simulink model "MARS"  (R2022a)
settings: Solver=VariableStepAuto  StartTime=0.0  StopTime=inf  RelTol=1e-3
model workspace (MAT data in the model file):
  T0 = -23.4
  h_trop = 7
  ingenuityParams : object (value not decoded)
values from neighbouring files (symbols this model uses):
  ingenuityParams =     [marsBatParam.mat]
undefined symbols (not defined in the file or in its folder): body, collective1, collective2, duration, ingenuity, leg1, leg2, leg3, leg4, link_name, model_name, rotor1, rotor2, solarPanel, world_pose
libraries: fl_lib x35, robotgazebolib x31, nesl_utility x12, ee_lib x11, slpidlib x3, sharedtransform x2, simulink x1, shared6dof x1, aerolibwind2 x1
(part 3 of 3)

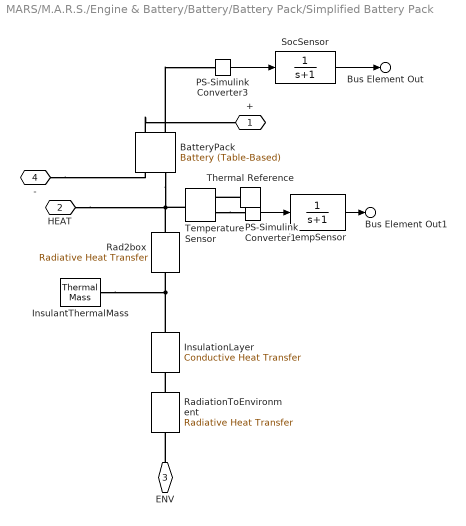
== system MARS/M.A.R.S./Engine & Battery/Battery/Battery Pack/Simplified Battery Pack ==
  BatteryPack : ee_lib/Sources/Battery (Table-Based)  SOC_vec=ingenuityParams.battery.cell.SOCvec  T_dependence=ee.enum.temperature_dependence.yes  prm_dir=ee.enum.battery.prm_dir.noCurrentDirectionality  T_vec=ingenuityParams.battery.cell.Tvec degC  V0_mat=ingenuityParams.battery.cell.V0_TLU*ingenuityParams.battery.numSeriesCells V  V0_vec=[3.1, 3.27, 3.31, 3.5] V  R0_mat=ingenuityParams.battery.cell.R0_TLU*ingenuityParams.battery.numSeriesCells/ingenuityParams.battery.numParallelStrings Ohm  R0_vec=[.015, .017, .012, .013] Ohm  R0_dis_mat=[.03, .015, .002; .04, .017, .008; .039, .012, .006; .027, .013, .021] Ohm  R0_dis_vec=[.015, .017, .012, .013] Ohm  R0_ch_mat=[.03, .015, .002; .04, .017, .008; .039, .012, .006; .027, .013, .021] Ohm  R0_ch_vec=[.015, .017, .012, .013] Ohm  AH=ingenuityParams.battery.cell.AH_TLU*ingenuityParams.battery.numParallelStrings A*hr  prm_leak=ee.enum.battery.prm_leak.disabled  Rleak_vec=[8000, 7000, 6000] Ohm  Rleak=7e3 Ohm  extrapolation_option=simscape.enum.extrapolation.nearest  SOC_port=ee.enum.enable.yes  V_range=[0, inf] V  prm_dyn=ee.enum.battery.prm_dyn.off  R1_mat=[.089, .076, .01; .042, .022, .099; .019, .007, .002; .051, .043, .029] Ohm  R1_vec=[.076, .022, .007, .043] Ohm  tau1_mat=[44, 148, 235; 93, 110, 1000; 19, 27, 133; .5, 22, 3] s  tau1_vec=[148, 110, 27, 22] s  R2_mat=[.014, .382, .407; .028, .006, .007; .014, .007, .006; .333, .956, .912] Ohm  R2_vec=[.382, .006, .007, .956] Ohm  tau2_mat=[1, 44, 5644; 11, 24, 506; 2, 14, 330; 3310, 13419, 30216] s  tau2_vec=[44, 24, 14, 13419] s  R3_mat=[.014, .382, .407; .028, .006, .007; .014, .007, .006; .333, .956, .912] Ohm  R3_vec=[.382, .006, .007, .956] Ohm  tau3_mat=[1, 44, 5644; 11, 24, 506; 2, 14, 330; 3310, 13419, 30216] s  tau3_vec=[44, 24, 14, 13419] s  R4_mat=[.014, .382, .407; .028, .006, .007; .014, .007, .006; .333, .956, .912] Ohm  R4_vec=[.382, .006, .007, .956] Ohm  tau4_mat=[1, 44, 5644; 11, 24, 506; 2, 14, 330; 3310, 13419, 30216] s  tau4_vec=[44, 24, 14, 13419] s  R5_mat=[.014, .382, .407; .028, .006, .007; .014, .007, .006; .333, .956, .912] Ohm  R5_vec=[.382, .006, .007, .956] Ohm  tau5_mat=[1, 44, 5644; 11, 24, 506; 2, 14, 330; 3310, 13419, 30216] s  tau5_vec=[44, 24, 14, 13419] s  prm_fade=ee.enum.battery.prm_fade.equations  N0=100  dV0=0  dR0=0  dAH=0  dRleak=0  dR1=0  dR2=0  dR3=0  dR4=0  dR5=0  N0vec=[100, 200, 300]  Tfadevec=[298.15, 323.15] K  dV0vec=[0, 0, 0]  dR0vec=[0, 0, 0]  dAHvec=[0, 0, 0]  dRleakvec=[0, 0, 0]  dR1vec=[0, 0, 0]  dR2vec=[0, 0, 0]  dR3vec=[0, 0, 0]  dR4vec=[0, 0, 0]  dR5vec=[0, 0, 0]  dV0mat=[0, 0; 0, 0; 0, 0]  dR0mat=[0, 0; 0, 0; 0, 0]  dAHmat=[0, 0; 0, 0; 0, 0]  dRleakmat=[0, 0; 0, 0; 0, 0]  dR1mat=[0, 0; 0, 0; 0, 0]  dR2mat=[0, 0; 0, 0; 0, 0]  dR3mat=[0, 0; 0, 0; 0, 0]  dR4mat=[0, 0; 0, 0; 0, 0]  dR5mat=[0, 0; 0, 0; 0, 0]  prm_age_modeling=ee.enum.battery.prm_age_modeling.equation  storage_dt_age_vec=[0] d  storage_T_age_vec=[273] K  prm_age_OCV=ee.enum.battery.prm_age_OCV.OCV  OCV_age=0.9  SOC_age=0.6  prm_age_resistance=ee.enum.battery.prm_age.disabled  OCV_scaling_age_resistance=2.2134e6  OCV_offset_age_resistance=1.632e6  temp_exp_age_resistance=0.515833569 V  t_exp_age_resistance=0.75  T_age_vec_resistance=[273.15, 298.15, 323.15] K  dt_age_vec_resistance=[90, 180, 270, 360] d  dR0_age_vec=[0, 0, 0]  t_meas_dR0_age=100 d  dR0_age_mat=[0, 0, 0; 0, 0, 0; 0, 0, 0; 0, 0, 0]  prm_age_capacity=ee.enum.battery.prm_age.disabled  OCV_scaling_age_capacity=1.5097e07  OCV_offset_age_capacity=8.3625e06  temp_exp_age_capacity=0.6011 V  t_exp_age_capacity=0.75  T_age_vec_capacity=[273.15, 298.15, 323.15] K  dt_age_vec_capacity=[90, 180, 270, 360] d  dAH_age_vec=[0, 0, 0]  t_meas_dAH_age=100 d  dAH_age_mat=[0, 0, 0; 0, 0, 0; 0, 0, 0; 0, 0, 0]  thermal_port=simscape.enum.thermaleffects.model  temperature=ingenuityParams.battery.cell.T_init degC  thermal_mass=ingenuityParams.battery.cell.mass*ingenuityParams.battery.cell.cp*ingenuityParams.battery.numCells J/K  i_specify=off  i_priority=None  i=0 A  i_nominal_specify=off  i_nominal_unit=A  i_nominal_value=1  v_specify=off  v_priority=None  v=0 V  v_nominal_specify=off  v_nominal_unit=V  v_nominal_value=1  stateOfCharge_specify=on  stateOfCharge_priority=High  stateOfCharge=ingenuityParams.battery.cell.SOC_init  stateOfCharge_nominal_specify=off  stateOfCharge_nominal_unit=1  stateOfCharge_nominal_value=1  num_cycles_specify=off  num_cycles_priority=High  num_cycles=0  num_cycles_nominal_specify=off  num_cycles_nominal_unit=1  num_cycles_nominal_value=1  cell_temperature_specify=on  cell_temperature_priority=High  cell_temperature=ingenuityParams.battery.cell.T_init degC  cell_temperature_nominal_specify=off  cell_temperature_nominal_unit=K  cell_temperature_nominal_value=1
      settings: SourceProductBaseCode=PS  LogSimulationData=on  InternalSimscapePortConfiguration="{\"Bottom\":[],\"Left\":[{\"id\":\"p\",\"label\":\"+\",\"type\":\"foundation.electrical.electrical\"},{\"id\":\"soc\",\"label\":\"SOC\",\"type\":\"output\"}],\"Right\":[{\"id\":\"n\",\"label\":\"-\",\"type\":\"foundation.electrical.electrical\"},{\"id\":\"H\",\"label\":\"H\",\"type\":\"foundation.thermal.thermal\"}],\"Top\":[]}"
  InsulantThermalMass : fl_lib/Thermal/Thermal Elements/Thermal Mass  mass=ingenuityParams.battery.thermal.insulantThermalMass.mass kg  sp_heat=ingenuityParams.battery.thermal.insulantThermalMass.cp J/kg/K  T_specify=on  T_priority=High  T=ingenuityParams.battery.cell.T_init degC  T_nominal_specify=off  T_nominal_unit=K  T_nominal_value=1  Q_specify=off  Q_priority=None  Q=0 W  Q_nominal_specify=off  Q_nominal_unit=W  Q_nominal_value=1
      settings: SourceProductBaseCode=PW,SS,VE  LogSimulationData=on
  InsulationLayer : fl_lib/Thermal/Thermal Elements/Conductive Heat Transfer  area=ingenuityParams.battery.thermal.insulationLayer.area m^2  thickness=ingenuityParams.battery.thermal.insulationLayer.thick m  th_cond=ingenuityParams.battery.thermal.insulationLayer.k W/(m*K)  T_specify=off  T_priority=None  T=0 K  T_nominal_specify=off  T_nominal_unit=K  T_nominal_value=1  Q_specify=off  Q_priority=None  Q=0 W  Q_nominal_specify=off  Q_nominal_unit=W  Q_nominal_value=1
      settings: SourceProductBaseCode=PW,SS,VE  LogSimulationData=on
  PS-Simulink Converter1 : nesl_utility/PS-Simulink Converter  PhysicalDomain=network_engine_domain  SubClassName=ps_output  LeftPortType=input  RightPortType=output  PseudoPeriodic=off  Frequencies=[]  VectorFormat=1-D array  Unit=degC  AffineConversion=on
      settings: SourceProductBaseCode=SS,PW,VE
  PS-Simulink Converter3 : nesl_utility/PS-Simulink Converter  PhysicalDomain=network_engine_domain  SubClassName=ps_output  LeftPortType=input  RightPortType=output  PseudoPeriodic=off  Frequencies=[]  VectorFormat=1-D array  Unit=1  AffineConversion=off
      settings: SourceProductBaseCode=SS,PW,VE
  Rad2box : fl_lib/Thermal/Thermal Elements/Radiative Heat Transfer  area=ingenuityParams.battery.thermal.radToBox.area*ingenuityParams.battery.numCells m^2  rad_tr_coeff=ingenuityParams.battery.thermal.radToBox.radCoeff W/(m^2*K^4)  T_specify=off  T_priority=None  T=0 K  T_nominal_specify=off  T_nominal_unit=K  T_nominal_value=1  Q_specify=off  Q_priority=None  Q=0 W  Q_nominal_specify=off  Q_nominal_unit=W  Q_nominal_value=1
      settings: SourceProductBaseCode=PW,SS,VE  LogSimulationData=on  InternalSimscapePortConfiguration="{\"Bottom\":[],\"Left\":[{\"id\":\"A\",\"label\":\"A\",\"type\":\"foundation.thermal.thermal\"}],\"Right\":[{\"id\":\"B\",\"label\":\"B\",\"type\":\"foundation.thermal.thermal\"}],\"Top\":[]}"
  RadiationToEnvironment : fl_lib/Thermal/Thermal Elements/Radiative Heat Transfer  area=ingenuityParams.battery.thermal.radToEnvironment.area m^2  rad_tr_coeff=ingenuityParams.battery.thermal.radToEnvironment.radCoeff W/(m^2*K^4)  T_specify=off  T_priority=None  T=0 K  T_nominal_specify=off  T_nominal_unit=K  T_nominal_value=1  Q_specify=off  Q_priority=None  Q=0 W  Q_nominal_specify=off  Q_nominal_unit=W  Q_nominal_value=1
      settings: SourceProductBaseCode=PW,SS,VE  LogSimulationData=on  InternalSimscapePortConfiguration="{\"Bottom\":[],\"Left\":[{\"id\":\"A\",\"label\":\"A\",\"type\":\"foundation.thermal.thermal\"}],\"Right\":[{\"id\":\"B\",\"label\":\"B\",\"type\":\"foundation.thermal.thermal\"}],\"Top\":[]}"
  SocSensor : TransferFcn  Denominator=[1 1]
  TempSensor : TransferFcn  Denominator=[1 1]
  Temperature Sensor : fl_lib/Thermal/Thermal Sensors/Temperature Sensor
      settings: SourceProductBaseCode=PW,SS,VE  LogSimulationData=on
  Thermal Reference : fl_lib/Thermal/Thermal Elements/Thermal Reference
      settings: SourceProductBaseCode=PW,SS,VE
  + : PMIOPort  Side=Left
  HEAT : PMIOPort  Port=2  Side=Right
  ENV : PMIOPort  Port=3  Side=Right
  - : PMIOPort  Port=4  Side=Right
  Bus Element Out : Outport  PortName=battery  Element=SOC3
  Bus Element Out1 : Outport  PortName=battery  Element=T3
  wires:
  SocSensor/1 -> Bus Element Out/1
  PS-Simulink Converter1/1 -> TempSensor/1
  PS-Simulink Converter3/1 -> SocSensor/1
  TempSensor/1 -> Bus Element Out1/1
  connections:
  InsulationLayer/LConn1 -- InsulantThermalMass/LConn1 -- Rad2box/RConn1
  BatteryPack/RConn2 -- Rad2box/LConn1 -- Temperature Sensor/LConn1 -- HEAT/RConn1
  BatteryPack/LConn2 -- PS-Simulink Converter3/LConn1
  RadiationToEnvironment/LConn1 -- InsulationLayer/RConn1
  ENV/RConn1 -- RadiationToEnvironment/RConn1
  BatteryPack/LConn1 -- +/RConn1
  Thermal Reference/LConn1 -- Temperature Sensor/RConn1
  Temperature Sensor/RConn2 -- PS-Simulink Converter1/LConn1
  -/RConn1 -- BatteryPack/RConn1

== stateflow chart MARS/M.A.R.S./Engine & Battery/System-Level Controls ==
  state Heating
    entry:
    heater = 1;
    fly = 0;
  state StandBy
    entry:
    heater = 0;
    fly = 0;
  state Land
    entry:
    heater = 0;
    fly = 1;
    during:
    altitudeRef = 0;
  state PrepareFlight
    entry:
    heater = 1;
    fly = 0;
  state Fly
    entry:
    heater = 0;
    fly = 1;
    during:
    altitudeRef = altitudeCom;
  (default) -> StandBy
  StandBy -> Heating [order 1] : [T < -15]
  Land -> StandBy : [altitude < 0.1]
  Heating -> StandBy : [T > -10 || SOC < 0.2]
  PrepareFlight -> StandBy [order 1] : [prepFlight == 0 || SOC <0.3]
  StandBy -> PrepareFlight [order 2] : [ prepFlight == 1 && SOC > 0.4]
  Fly -> Land : [prepFlight == 0 || SOC <0.3]
  PrepareFlight -> Fly [order 2] : [T>10]
  data: altitudeCom input; T input; SOC input; prepFlight input; heater output double; fly output; altitudeRef output; altitude input
